simulink subsystem "QRDecompose"  (R2023b)
settings: Solver=VariableStepAuto  StartTime=0.0  StopTime=10.0  RelTol=1e-3
values from neighbouring files (symbols this model uses):
  FrameLength = 260    [CustomQRMode.m]
undefined symbols (not defined in the file or in its folder): NumOfAntennas
libraries: dspstat3 x1
settings Model: Creator=Koche  LastModifiedBy=Koche

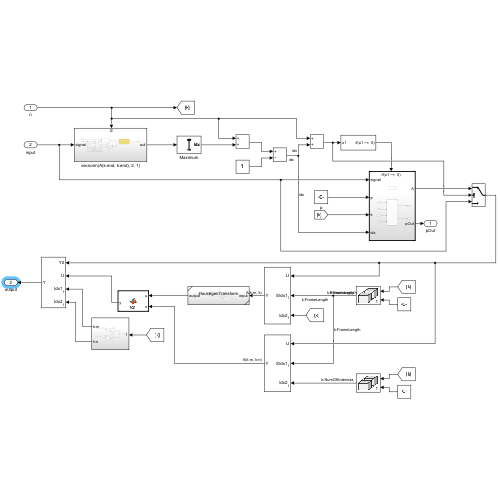
[thumbnail: Simulink's stored preview of the top-level diagram]
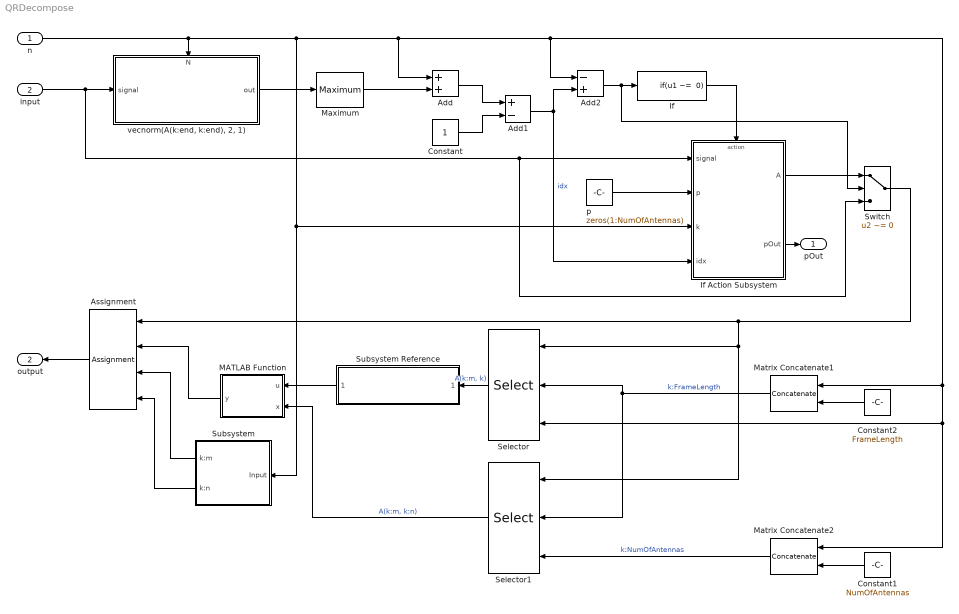
== system QRDecompose ==
  n : Inport
  input : Inport  Port=2
  Add : Sum
  Add1 : Sum  Inputs=+-
  Add2 : Sum  Inputs=-+
  Assignment : Assignment  NumberOfDimensions=2  IndexOptions=Index vector (port),Index vector (port)  Indices=1,1  OutputSizes=1,1
  Constant : Constant  SampleTime=-1
  Constant1 : Constant  Value=NumOfAntennas  OutDataTypeStr=int32  SampleTime=-1
  Constant2 : Constant  Value=FrameLength  OutDataTypeStr=int32  SampleTime=-1
  If : If  IfExpression="u1 ~=  0"  ShowElse=off
  If Action Subsystem : Subsystem  TreatAsAtomicUnit=on
  MATLAB Function : MATLAB Function  TreatAsAtomicUnit=on
  Matrix Concatenate1 : Concatenate  Mode=Multidimensional array
  Matrix Concatenate2 : Concatenate  Mode=Multidimensional array
  Maximum : dspstat3/Maximum  operation=maximum  fcn=Index  indexBase=One  operateOver=Each column  Dimension=1  InputProcessing=Columns as channels (frame based)  reset=None  roiEnable=off  roiType=Rectangles  roiPortion=Entire ROI  roiOutput=Individual statistics for each ROI  roiFlag=off  roundingMode=Floor  overflowMode=off  accumDataTypeStr=Inherit: Same as product output  accumLastDataTypeStr=Inherit: Same as product output
      settings: LibrarySourceBlock=dsphdlsupportstat/Maximum
  Selector : Selector  NumberOfDimensions=2  InputPortWidth=3  IndexOptions=Starting and ending indices (port),Index vector (port)  Indices=[1 3],1  OutputSizes=1,1
  Selector1 : Selector  NumberOfDimensions=2  InputPortWidth=3  IndexOptions=Starting and ending indices (port),Starting and ending indices (port)  Indices=[1 3],1  OutputSizes=1,1
  Subsystem : Subsystem
  Subsystem Reference : Subsystem  ReferencedSubsystem=HousegenTransform
  Switch : Switch  Criteria=u2 ~= 0  SaturateOnIntegerOverflow=off  InputSameDT=off
  p : Constant  Value=zeros(1:NumOfAntennas)  SampleTime=-1
  "vecnorm(A(k:end, k:end), 2, 1)" : Subsystem
      settings: PortSchema="{\"entries\":[{\"content\":{\"sides\":[{\"content\":{\"connectorIds\":[\"In1\"]},\"type\":\"ConnectorPlacement.EquallySpacedRectSide\",\"uuid\":\"ddbbb4e8-2c6c-4e6c-8e2e-3b3671634aad\"},{\"content\":{\"connectorIds\":[\"Out1\"],\"side\":\"RIGHT\"},\"type\":\"ConnectorPlacement.EquallySpacedRectSide\",\"uuid\":\"1781eb83-3214-4f0b-a111-2b3a2e27c9fb\"},{\"content\":{\"connectorIds\":[\"In2\"],\"side\":\"TOP\"},\"type\":\"ConnectorPlacement.EquallySpacedRectSide\",\"uuid\":\"ba31d641-ff62-4171-b945-e5cde8a84090\"}]},\"type\":\"ConnectorPlacement.EquallySpacedConnector\",\"uuid\":\"97f7897c-1f2b-447f-863d-894b57bebce4\"}],\"packageUris\":[\"http://schema.mathworks.com/mf0/Connector/R2020b\"],\"version\":\"1.0\"}"
  pOut : Outport
  output : Outport  Port=2
  wires:
  Subsystem Reference/1 -> MATLAB Function/1(u)
  Switch/1 -> Assignment/1, Selector1/1, Selector/1
  Add/1 -> Add1/1
  p/1 -> If Action Subsystem/2(p)
  Subsystem/1(k:m) -> Assignment/3
  Matrix Concatenate2/1 -> Selector1/3  "k:NumOfAntennas"
  MATLAB Function/1(y) -> Assignment/2
  If/1 -> If Action Subsystem/Action
  If Action Subsystem/1(A) -> Switch/1
  Constant2/1 -> Matrix Concatenate1/2
  "vecnorm(A(k:end, k:end), 2, 1)"/1(out) -> Maximum/1
  Add1/1 -> Add2/2, If Action Subsystem/4(idx)  "idx"
  Constant/1 -> Add1/2
  Selector/1 -> Subsystem Reference/1  "A(k:m, k)"
  Matrix Concatenate1/1 -> Selector1/2, Selector/2  "k:FrameLength"
  n/1 -> "vecnorm(A(k:end, k:end), 2, 1)"/2(N), Subsystem/1(Input), If Action Subsystem/3(k), Add/1, Add2/1, Matrix Concatenate1/1, Matrix Concatenate2/1, Selector/3
  If Action Subsystem/2(pOut) -> pOut/1
  Selector1/1 -> MATLAB Function/2(x)  "A(k:m, k:n)"
  Add2/1 -> If/1, Switch/2
  input/1 -> "vecnorm(A(k:end, k:end), 2, 1)"/1(signal), If Action Subsystem/1(signal), Switch/3
  Assignment/1 -> output/1
  Subsystem/2(k:n) -> Assignment/4
  Constant1/1 -> Matrix Concatenate2/2
  Maximum/1 -> Add/2

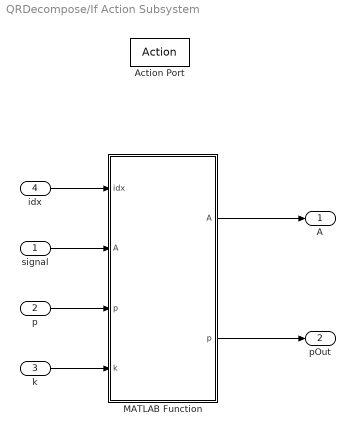
== system QRDecompose/If Action Subsystem ==
  signal : Inport
  p : Inport  Port=2
  k : Inport  Port=3
  idx : Inport  Port=4
  Action Port : ActionPort
  MATLAB Function : MATLAB Function  TreatAsAtomicUnit=on
  A : Outport
  pOut : Outport  Port=2
  wires:
  MATLAB Function/2(p) -> pOut/1
  MATLAB Function/1(A) -> A/1
  idx/1 -> MATLAB Function/1(idx)
  k/1 -> MATLAB Function/4(k)
  p/1 -> MATLAB Function/3("p ")
  signal/1 -> MATLAB Function/2("A ")

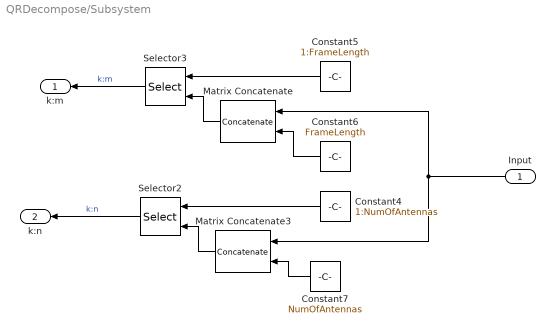
== system QRDecompose/Subsystem ==
  Input : Inport
  Constant4 : Constant  Value=1:NumOfAntennas  OutDataTypeStr=int32  SampleTime=-1
  Constant5 : Constant  Value=1:FrameLength  OutDataTypeStr=int32  SampleTime=-1
  Constant6 : Constant  Value=FrameLength  OutDataTypeStr=int32
  Constant7 : Constant  Value=NumOfAntennas  OutDataTypeStr=int32
  Matrix Concatenate : Concatenate  Mode=Multidimensional array
  Matrix Concatenate3 : Concatenate  Mode=Multidimensional array
  Selector2 : Selector  IndexOptions=Starting and ending indices (port)  Indices=[1 3]  OutputSizes=1
  Selector3 : Selector  IndexOptions=Starting and ending indices (port)  Indices=[1 3]  OutputSizes=1
  k:m : Outport
  k:n : Outport  Port=2
  wires:
  Input/1 -> Matrix Concatenate3/1, Matrix Concatenate/1
  Selector3/1 -> k:m/1  "k:m"
  Selector2/1 -> k:n/1  "k:n"
  Constant6/1 -> Matrix Concatenate/2
  Matrix Concatenate/1 -> Selector3/2
  Constant7/1 -> Matrix Concatenate3/2
  Constant4/1 -> Selector2/1
  Matrix Concatenate3/1 -> Selector2/2
  Constant5/1 -> Selector3/1

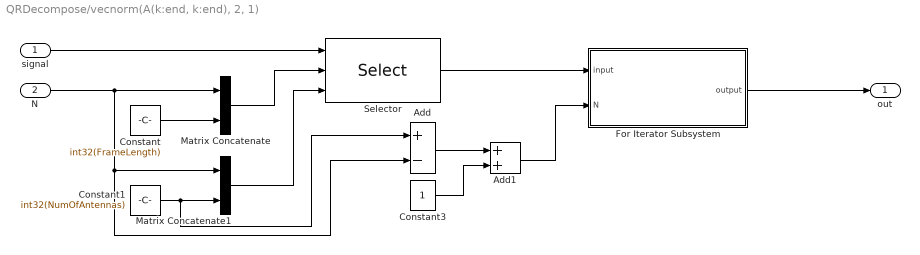
== system QRDecompose/vecnorm(A(k:end, k:end), 2, 1) ==
  signal : Inport
  N : Inport  Port=2
  Add : Sum  Inputs=+-
  Add1 : Sum
  Constant : Constant  Value=int32(FrameLength)  SampleTime=-1
  Constant1 : Constant  Value=int32(NumOfAntennas)  SampleTime=-1
  Constant3 : Constant
  For Iterator Subsystem : Subsystem  TreatAsAtomicUnit=on
  Matrix Concatenate : Concatenate
  Matrix Concatenate1 : Concatenate
  Selector : Selector  NumberOfDimensions=2  InputPortWidth=3  IndexOptions=Starting and ending indices (port),Starting and ending indices (port)  Indices=[1 3],1  OutputSizes=1,1
  out : Outport
  wires:
  Selector/1 -> For Iterator Subsystem/1(input)
  Add1/1 -> For Iterator Subsystem/2(N)
  For Iterator Subsystem/1(output) -> out/1
  Constant3/1 -> Add1/2
  Add/1 -> Add1/1
  N/1 -> Matrix Concatenate/1, Add/2, Matrix Concatenate1/1
  Constant1/1 -> Matrix Concatenate1/2, Add/1
  Matrix Concatenate1/1 -> Selector/3
  Constant/1 -> Matrix Concatenate/2
  Matrix Concatenate/1 -> Selector/2
  signal/1 -> Selector/1

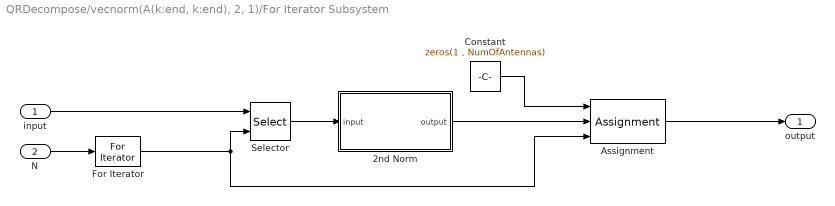
== system QRDecompose/vecnorm(A(k:end, k:end), 2, 1)/For Iterator Subsystem ==
  input : Inport
  N : Inport  Port=2
  2nd Norm : Subsystem
  Assignment : Assignment  IndexOptions=Index vector (port)  Indices=1  OutputSizes=1
  Constant : Constant  Value=zeros(1 , NumOfAntennas)
  For Iterator : ForIterator  ResetStates=reset  IterationSource=external
  Selector : Selector  NumberOfDimensions=2  InputPortWidth=3  IndexOptions=Select all,Index vector (port)  Indices=[1 3],1  OutputSizes=1,1
  output : Outport
  wires:
  Assignment/1 -> output/1
  2nd Norm/1(output) -> Assignment/2
  Constant/1 -> Assignment/1
  N/1 -> For Iterator/1
  Selector/1 -> 2nd Norm/1(input)
  For Iterator/1 -> Selector/2, Assignment/3
  input/1 -> Selector/1

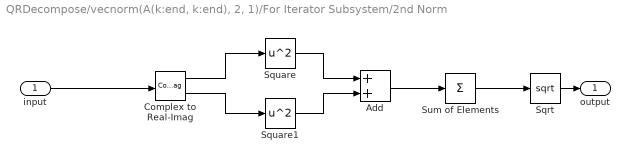
== system QRDecompose/vecnorm(A(k:end, k:end), 2, 1)/For Iterator Subsystem/2nd Norm ==
  input : Inport
  Add : Sum
  Complex to Real-Imag : ComplexToRealImag
  Sqrt : Sqrt
  Square : Math  Operator=square  SignedPower=on  RndMeth=Zero
  Square1 : Math  Operator=square  SignedPower=on  RndMeth=Zero
  Sum of Elements : Sum  Inputs=+
  output : Outport
  wires:
  input/1 -> Complex to Real-Imag/1
  Complex to Real-Imag/2 -> Square1/1
  Sqrt/1 -> output/1
  Complex to Real-Imag/1 -> Square/1
  Square/1 -> Add/1
  Add/1 -> Sum of Elements/1
  Sum of Elements/1 -> Sqrt/1
  Square1/1 -> Add/2

== matlab function QRDecompose/If Action Subsystem/MATLAB Function ==
  data: idx input; A input; A output; p input; k input; p output
function [A, p] = swap(idx , A , p , k )
%#codegen
    A(:, [k, idx]) = A(:, [idx, k]);
    p([k, idx]) = p([idx, k]);
end

== matlab function QRDecompose/MATLAB Function ==
  data: u input; y output size=[260 4]; x input
function y = fcn(u, x)
    y = x - u*(u'*x);
end
